simulink model "auto_lights"  (R2019b)
settings: Solver=FixedStepDiscrete  StartTime=0.0  StopTime=inf  RelTol=1e-3
undefined symbols (not defined in the file): green_locked, green_requested, GREENDELAY, MAXREDDELAY, MINGREENDELAY, REDDELAY, YELLOWDELAY
libraries: sf_traffic_light_lib x2
settings Model: Creator=venka  LastModifiedBy=venka

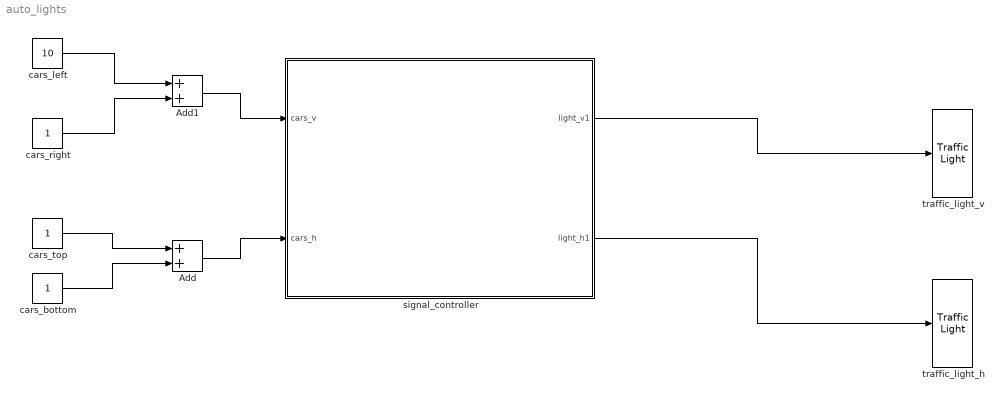
== system auto_lights ==
  Add : Sum
  Add1 : Sum
  cars_bottom : Constant
  cars_left : Constant  Value=10
  cars_right : Constant
  cars_top : Constant
  signal_controller : Stateflow chart  BlockKeywords=__PRM__SERIALIZED__DATA__:Stateflow Chart,Stateflow Diagram  TreatAsAtomicUnit=on  mask{Parameter1=6, Parameter2=180, Parameter3=15, Parameter4=120, Parameter5=360}
      mask prompts: Parameter1 "REDDELAY"; Parameter2 "GREENDELAY"; Parameter3 "YELLOWDELAY"; Parameter4 "MINGREENDELAY"; Parameter5 "MAXREDDELAY"
  traffic_light_h : sf_traffic_light_lib/Traffic Light  mode=LightModeType.Red
  traffic_light_v : sf_traffic_light_lib/Traffic Light  mode=LightModeType.Red
  wires:
  cars_right/1 -> Add1/2
  cars_left/1 -> Add1/1
  cars_top/1 -> Add/1
  cars_bottom/1 -> Add/2
  Add1/1 -> signal_controller/1(cars_v)
  Add/1 -> signal_controller/2(cars_h)
  signal_controller/1(light_v1) -> traffic_light_v/1
  signal_controller/2(light_h1) -> traffic_light_h/1

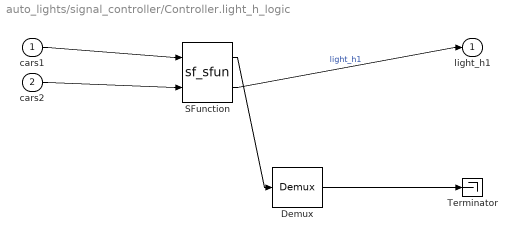
== system auto_lights/signal_controller/Controller.light_h_logic ==
  cars1 : Inport
  cars2 : Inport  Port=2
  " Demux " : Demux  Outputs=1
  " SFunction " : S-Function  Tag=Stateflow S-Function 2  FunctionName=sf_sfun  Parameters=GREENDELAY,MAXREDDELAY,MINGREENDELAY,REDDELAY,YELLOWDELAY  PortCounts=[2 2]  SFunctionDeploymentMode=off  EnableBusSupport=off
  " Terminator " : Terminator
  light_h1 : Outport
  wires:
  cars1/1 -> " SFunction "/1
  cars2/1 -> " SFunction "/2
  " SFunction "/2 -> light_h1/1  "light_h1"
  " Demux "/1 -> " Terminator "/1
  " SFunction "/1 -> " Demux "/1

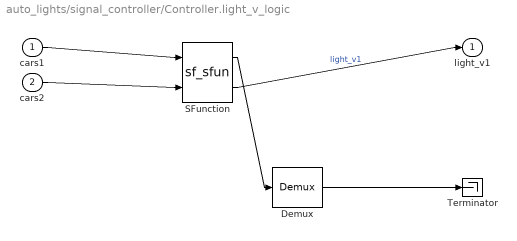
== system auto_lights/signal_controller/Controller.light_v_logic ==
  cars1 : Inport
  cars2 : Inport  Port=2
  " Demux " : Demux  Outputs=1
  " SFunction " : S-Function  Tag=Stateflow S-Function 1  FunctionName=sf_sfun  Parameters=GREENDELAY,MAXREDDELAY,MINGREENDELAY,REDDELAY,YELLOWDELAY  PortCounts=[2 2]  SFunctionDeploymentMode=off  EnableBusSupport=off
  " Terminator " : Terminator
  light_v1 : Outport
  wires:
  cars1/1 -> " SFunction "/1
  cars2/1 -> " SFunction "/2
  " SFunction "/2 -> light_v1/1  "light_v1"
  " Demux "/1 -> " Terminator "/1
  " SFunction "/1 -> " Demux "/1

== stateflow chart auto_lights/signal_controller/Controller.light_v_logic ==
  state RED
    state DELAY
    state WaitForInput
    state WaitUntilSafeToChange
      green_requested=true;
    (default) -> DELAY
    WaitForInput -> WaitUntilSafeToChange [order 2] : [after(MAXREDDELAY,sec)]
    DELAY -> WaitForInput : [after(REDDELAY,sec)]
    WaitForInput -> WaitUntilSafeToChange [order 1] : [cars1>cars2]
  state GREEN
    green_locked=true;
    green_requested=false;
  state YELLOW
    green_locked=false;
  (default) -> RED
  YELLOW -> RED : [after(YELLOWDELAY,sec)]
  RED -> GREEN : [after(REDDELAY,sec) && ~green_locked]
  GREEN -> YELLOW [order 1] : [after(GREENDELAY,sec)]
  GREEN -> YELLOW [order 2] : [after(MINGREENDELAY,sec) && green_requested]
  data: cars1 input; cars2 input; green_locked data_store_memory; green_requested data_store_memory; GREENDELAY parameter; REDDELAY parameter; YELLOWDELAY parameter; MAXREDDELAY parameter; MINGREENDELAY parameter; light_v1 output

== stateflow chart auto_lights/signal_controller/Controller.light_h_logic ==
  state RED
    state DELAY
    state WaitForInput
    state WaitUntilSafeToChange
      green_requested=true;
    (default) -> DELAY
    WaitForInput -> WaitUntilSafeToChange [order 2] : [after(MAXREDDELAY,sec)]
    DELAY -> WaitForInput : [after(REDDELAY,sec)]
    WaitForInput -> WaitUntilSafeToChange [order 1] : [cars1>cars2]
  state GREEN
    green_locked=true;
    green_requested=false;
  state YELLOW
    green_locked=false;
  (default) -> RED
  YELLOW -> RED : [after(YELLOWDELAY,sec)]
  RED -> GREEN : [after(REDDELAY,sec) && ~green_locked]
  GREEN -> YELLOW [order 1] : [after(GREENDELAY,sec)]
  GREEN -> YELLOW [order 2] : [after(MINGREENDELAY,sec) && green_requested]
  data: cars1 input; cars2 input; green_locked data_store_memory; green_requested data_store_memory; GREENDELAY parameter; REDDELAY parameter; YELLOWDELAY parameter; MAXREDDELAY parameter; MINGREENDELAY parameter; light_h1 output

== stateflow chart auto_lights/signal_controller ==
  state Controller
    state light_v_logic [parallel]
      settings: executionOrder=1
    state light_h_logic [parallel]
      settings: executionOrder=2
  (default) -> Controller
  data: cars_v input; cars_h input; green_locked local boolean; green_requested local boolean; light_v1 output Enum: LightModeType; light_h1 output Enum: LightModeType; REDDELAY parameter; YELLOWDELAY parameter; MINGREENDELAY parameter; GREENDELAY parameter; MAXREDDELAY parameter
